simulink model "IPmodel_SS"  (Simulink 7.1)
settings: Solver=ode1  StartTime=0.0  StopTime=5  FixedStep=0.001  RelTol=1e-3
PostLoadFcn:
  | , if any(exist('dsrtsu_mdlpostloadfcn', 'file') == [2, 3, 6]), try dsrtsu_mdlpostloadfcn('Execute', bdroot); catch fprintf('Error in PostLoadFcn (dsrtsu_mdlpostloadfcn) for model "%s":\n %s\n', bdroot, lasterr); end, end,
settings Model: Creator=atdummy  LastModifiedBy=Jian  BufferReuse=off  RTILINMMDATA=struct('GeneralSetupData',[])  DSRTSU_INTERNAL_RTI_VER=330  DSRTSU_INTERNAL_RTI_TYPE=rti1401
settings OptimizationCC: BlockReduction=off  OptimizeBlockIOStorage=off  BufferReuse=off  ExpressionFolding=off  LocalBlockOutputs=off
settings DebuggingCC: SaveWithParameterizedLinksMsg=none
settings HardwareCC: ProdIntDivRoundTo=Zero  ProdEndianess=BigEndian  ProdHWDeviceType=Specified  TargetIntDivRoundTo=Zero  TargetEndianess=BigEndian
settings RTWCC: SystemTargetFile=rti1401.tlc  MakeCommand=make_rti  TemplateMakefile=rti1401.tmf  Description=dSPACE DS1401 Hardware Platform  ProcessScript=rti1401_make_rtw_hook
settings STFCustomTargetCC: TargetFcnLib=ansi_tfl_tmw.mat  MatFileLogging=on  SystemTargetFile=rti1401.tlc
settings GRTTargetCC: TargetFcnLib=ansi_tfl_tmw.mat  CompOptLevelCompliant=off  ExtModeMexFile=noextcomm
settings CustomProperty: DataType=RTWOptions_EnumType_C__dSPACE_matlab_rti1401_tlc_rti1401_InitialSimState  Value=RUN
settings EnumStrPairs: String=RUN

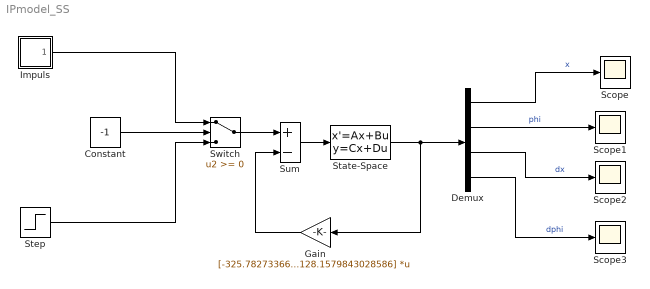
== system IPmodel_SS ==
  Constant : Constant  Value=-1  OutDataType=sfix(16)  OutScaling=2^0
  Demux : Demux
  Gain : Gain  Orientation=left  Gain=[-325.7827336669318 -621.9414030984024 -195.37905842480814 -128.1579843028586]  Multiplication=Matrix(K*u)  ParameterDataType=sfix(16)  ParameterScaling=2^0  OutDataType=sfix(16)  OutScaling=2^0
  "Impuls " : Subsystem  mask(Impulse Generator){T=1, dt=0.001, V=1}
      mask prompts: T "Impulse Time"; dt "Impulse Duration"; V "Finalvalue"
      mask help: This model generates an impulse of specified width.
      mask Help: This model generates an impulse of specified width.
      mask Display: plot(0,0,8,4,[1 2 3 4 4 4 5 6 7],[1 1 1 1 3 1 1 1 1])
  Scope{,1..3} (4 alike) : Scope
      Scope2 settings: SaveName=ScopeData2
      Scope3 settings: SaveName=ScopeData3
  State-Space : StateSpace  A=[0 0 1 0;0 0 0 1; 0 -0.88 -1.915 0.0056; 0 21.473 3.85 -0.136]  B=[0;0;0.30882;-0.62032]  C=[1 0 0 0;0 1 0 0;0 0 1 0;0 0 0 1]  D=[0;0;0;0]
  Step : Step  SampleTime=0
  Sum : Sum  Inputs=+-  OutDataType=sfix(16)  OutScaling=2^0
  Switch : Switch
  wires:
  State-Space/1 -> Gain/1, Demux/1
  Sum/1 -> State-Space/1
  Gain/1 -> Sum/2
  Demux/1 -> Scope/1  "x"
  Demux/2 -> Scope1/1  "phi"
  Demux/3 -> Scope2/1  "dx"
  Demux/4 -> Scope3/1  "dphi"
  "Impuls "/1(Impulse) -> Switch/1
  Switch/1 -> Sum/1
  Step/1 -> Switch/3
  Constant/1 -> Switch/2

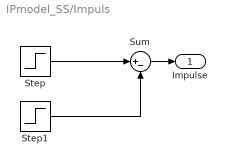
== system IPmodel_SS/Impuls  ==
  Step : Step  Time=T  After=V  SampleTime=0
  Step1 : Step  Time=T + dt  After=V  SampleTime=0
  Sum : Sum  Inputs=|+-  OutDataType=sfix(16)  OutScaling=2^0  SaturateOnIntegerOverflow=on  InputSameDT=on  OutDataTypeStr=Inherit: Same as first input
  Impulse : Outport
  wires:
  Step/1 -> Sum/1
  Step1/1 -> Sum/2
  Sum/1 -> Impulse/1
